simulink model "SimpleDynamicsModel"  (R2020a)
settings: Solver=VariableStepAuto  StartTime=0.0  StopTime=5  RelTol=1e-3
values from neighbouring files (symbols this model uses):
  b = 0.0015    [parameters.m]
  c = 0.02    [parameters.m]
  Fa = Famax    (= 80)    [parameters.m]
  Fb = 0    [parameters.m]
  m = 13    [parameters.m]
  v0 = 0    [parameters.m]
  x0 = 0    [parameters.m]
settings Model: SimulationMode=rapid-accelerator  Creator=bertu  LastModifiedBy=bertu

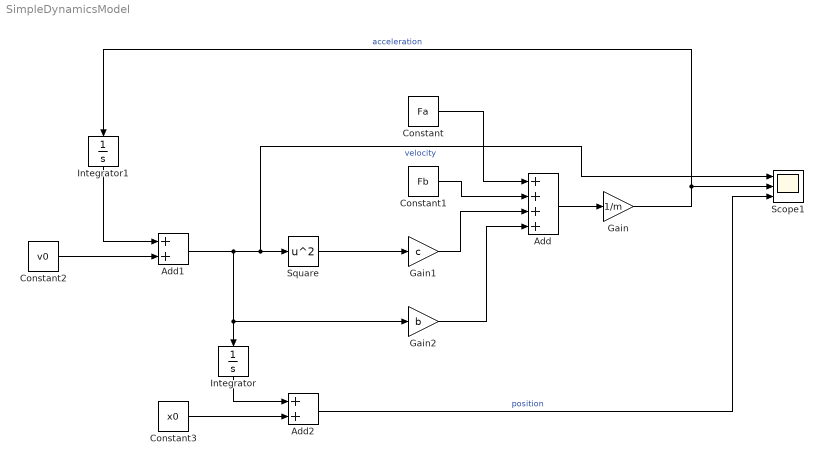
== system SimpleDynamicsModel ==
  Add : Sum  Inputs=++++
  Add1 : Sum
  Add2 : Sum
  Constant : Constant  Value=Fa
  Constant1 : Constant  Value=Fb
  Constant2 : Constant  Value=v0
  Constant3 : Constant  Value=x0
  Gain : Gain  Gain=1/m
  Gain1 : Gain  Gain=c
  Gain2 : Gain  Gain=b
  Integrator : Integrator
  Integrator1 : Integrator
  Scope1 : Scope  NumInputPorts=3
  Square : Math  Operator=square  SaturateOnIntegerOverflow=on
  wires:
  Constant/1 -> Add/1
  Constant1/1 -> Add/2
  Gain1/1 -> Add/3
  Gain2/1 -> Add/4
  Square/1 -> Gain1/1
  Add1/1 -> Integrator/1, Gain2/1, Scope1/1, Square/1  "velocity"
  Constant2/1 -> Add1/2
  Integrator/1 -> Add2/1
  Constant3/1 -> Add2/2
  Integrator1/1 -> Add1/1
  Add/1 -> Gain/1
  Gain/1 -> Scope1/2, Integrator1/1  "acceleration"
  Add2/1 -> Scope1/3  "position"
